simulink model "vision_try_3_old"  (R2016b)
settings: Solver=VariableStepAuto  StartTime=0.0  StopTime=inf  RelTol=1e-3
undefined symbols (not defined in the file): gray
libraries: visiontextngfix x1, dspvision x1, visionanalysis x1
settings Model: Creator=bhawnath.tiwari  LastModifiedBy=bhawnath.tiwari

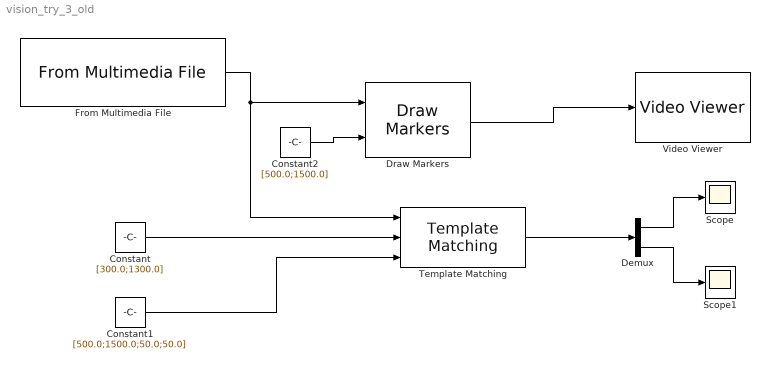
== system vision_try_3_old ==
  Constant : Constant  Value=[300.0;1300.0]  OutDataTypeStr=single
  Constant1 : Constant  Value=[500.0;1500.0;50.0;50.0]  OutDataTypeStr=single
  Constant2 : Constant  Value=[500.0;1500.0]  OutDataTypeStr=single
  Demux : Demux  Outputs=2
  Draw Markers : visiontextngfix/Draw Markers  shape=Square  size=300  fill=off  fillClrSource=Specify via dialog  display=Black  intensity=200  color=[200 255 100]  opacity=0.6  viewport=Entire image  antialiasing=off  inType=Obsolete  imagePorts=One multidimensional signal  prodOutputMode=Binary point scaling  prodOutputWordLength=32  prodOutputFracLength=14  memoryMode=Specify word length  memoryWordLength=16  memoryFracLength=15  roundingMode=Floor  overflowMode=off
  From Multimedia File : dspvision/From Multimedia File  inputFilename=G:\Utilisateurs\bhawnath.tiwari\Documents\MATLAB\testr1.avi  loop=on  numPlays=inf  outputStreams=Video only  videoDataType=single  audioDataType=int16  inheritSampleTime=on  userDefinedSampleTime=1/30  noAudioOutput=off  isIntensityVideo=off  fourcc=Intensity  colorVideoFormat=One multidimensional signal  outputEOF=off  dataOrg=Column-major  audioFrameSize=1024  computeAudioFrameSize=off  outSamplingMode=Sample based
  Scope : Scope
  Scope1 : Scope
  Template Matching : visionanalysis/Template Matching  metric=Sum of absolute differences  output=Best match location  method=Exhaustive  nMetric=off  nSize=3  roi=on  roiValid=off  accumMode=Binary point scaling  accumWordLength=32  accumFracLength=0  prodOutputMode=Binary point scaling  prodOutputWordLength=32  prodOutputFracLength=0  roundingMode=Floor  overflowMode=off
  Video Viewer : VideoViewer  colormapValue=gray(256)  FigPos=[1 1038 1920 938]
  wires:
  From Multimedia File/1 -> Draw Markers/1, Template Matching/1
  Constant/1 -> Template Matching/2
  Constant1/1 -> Template Matching/3
  Template Matching/1 -> Demux/1
  Demux/1 -> Scope/1
  Demux/2 -> Scope1/1
  Constant2/1 -> Draw Markers/2
  Draw Markers/1 -> Video Viewer/1
